simulink model "Aizawa"  (R2014b)
settings: Solver=ode45  StartTime=0.0  StopTime=10.0  RelTol=1e-3
values from neighbouring files (symbols this model uses):
  a = 0.95    [Run_Aizawa.m]    (also in Run_Arneodo.m = -5.5; Run_Chen.m = 33; Run_Chua.m = 15.6; Run_Chua_4D.m = 0.03)
  b = 0.7    [Run_Aizawa.m]    (also in Run_Arneodo.m = 3.5; Run_Chen.m = 3; Run_Chua.m = 28; Run_Duffing.m = 100)
  g = 0.65    [Run_Aizawa.m]    (also in Run_RabinovichFabrikant.m = 0.09)
  s = 3.5    [Run_Aizawa.m]    (also in Run_Chua_4D.m = 0.75; Run_Duffing.m = 0.2; Run_HindmarshRose.m = 4; Run_Lorenz.m = 10)
undefined symbols (not defined in the file or in its folder): param
settings Model: Creator=Arek  LastModifiedBy=Arek

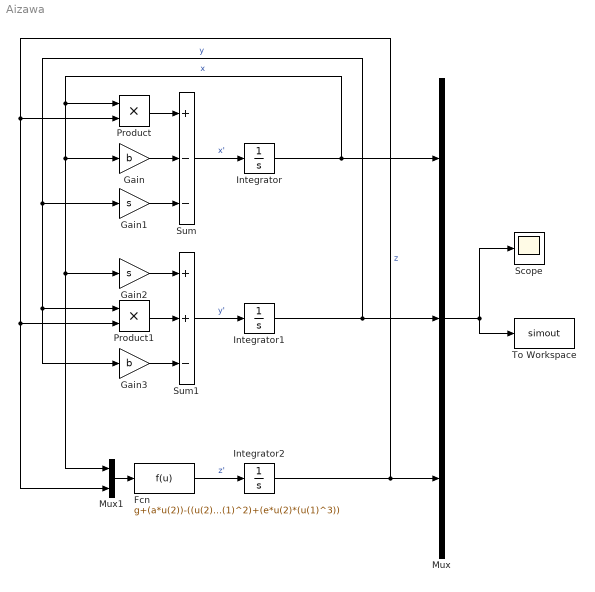
== system Aizawa ==
  Fcn : Fcn  Expr=g+(a*u(2))-((u(2)^3)/3)-(u(1)^2)+(e*u(2)*(u(1)^3))
  Gain : Gain  Gain=b
  Gain1 : Gain  Gain=s
  Gain2 : Gain  Gain=s
  Gain3 : Gain  Gain=b
  Integrator : Integrator  InitialCondition=param.ic(1)
  Integrator1 : Integrator  InitialCondition=param.ic(2)
  Integrator2 : Integrator  InitialCondition=param.ic(3)
  Mux : Mux  Inputs=3
  Mux1 : Mux  Inputs=2
  Product : Product
  Product1 : Product
  Scope : Scope
      settings: ShowLegends=on
  Sum : Sum  Inputs=+--
  Sum1 : Sum  Inputs=++-
  To Workspace : ToWorkspace  VariableName=simout  SaveFormat=Timeseries  SampleTime=-1
  wires:
  Integrator/1 -> Product/1, Mux1/1, Gain2/1, Gain/1, Mux/1  "x"
  Sum1/1 -> Integrator1/1  "y'"
  Integrator1/1 -> Gain3/1, Product1/1, Gain1/1, Mux/2  "y"
  Fcn/1 -> Integrator2/1  "z'"
  Integrator2/1 -> Product/2, Mux1/2, Product1/2, Mux/3  "z"
  Mux/1 -> Scope/1, To Workspace/1
  Sum/1 -> Integrator/1  "x'"
  Product/1 -> Sum/1
  Gain/1 -> Sum/2
  Gain1/1 -> Sum/3
  Gain3/1 -> Sum1/3
  Gain2/1 -> Sum1/1
  Product1/1 -> Sum1/2
  Mux1/1 -> Fcn/1
